simulink model "MPPT_pv_system"  (R2020a)
settings: Solver=VariableStepAuto  StartTime=0.0  StopTime=1  RelTol=1e-3
libraries: powerlib x18, re_lib x1, simulink x1
settings Model: Creator=hp  LastModifiedBy=hp

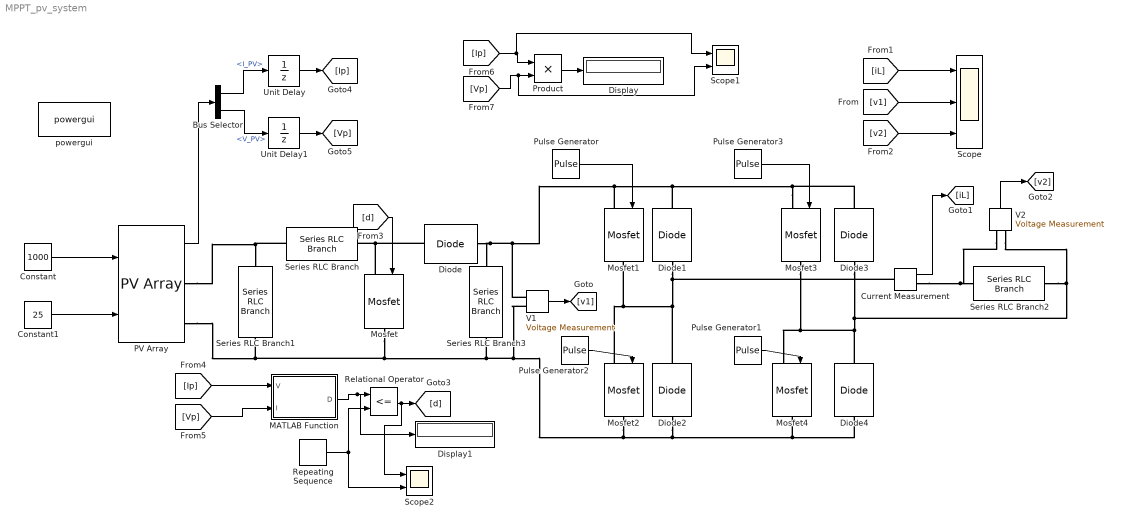
== system MPPT_pv_system ==
  Bus Selector : BusSelector  OutputSignals=I_PV,V_PV
  Constant : Constant  Value=1000
  Constant1 : Constant  Value=25
  Current Measurement : powerlib/Measurements/Current Measurement  PhasorSimulation=off  OutputType=Complex  PSBequivalent=0
  Diode{,1..4} (5 alike) : powerlib/Power Electronics/Diode  Ron=0.001  Lon=0  Vf=0.8  IC=0  UseSnubber=0  Rs=500  Cs=250e-9  Measurements=off
  Display : Display
  Display1 : Display
  MATLAB Function : MATLAB Function  TreatAsAtomicUnit=on
  Mosfet{,1..4} (5 alike) : powerlib/Power Electronics/Mosfet  Ron=0.1  Lon=0  Rd=0.01  Vfd=0  IC=0  Rs=1e5  Cs=inf  Measurements=off
  PV Array : re_lib/Solar/PV Array  Npar=4  Nser=4  PlotType=array @ 25 deg.C & specified irradiances  S_vec="[ 1000  500  100 ]"  Temp_C_vec="[ 45 25  ]"  ModuleName=Centrosolar America BP7-315BW  PlotWhenSelected=off  Pm=315.0042  Ncell=72  Voc=45.45  Isc=8.97  Vm=37.59  Im=8.38  beta_Voc_pc=-0.349  alpha_Isc_pc=0.037001  beta_Voc=-0.15862  alpha_Isc=0.003319  IL=8.9803  I0=1.9823e-10  nI=1.0022  Rsh=237.0635  Rs=0.27147  RobustModel=off  RobustCellTemperature=25  BAL=on  Tc=1e-6  Tfilter=5e-5
  Product : Product
  Pulse Generator : DiscretePulseGenerator  PulseType=Time based  Period=1/(50)  PulseWidth=50  PhaseDelay=0/(360*50)
  Pulse Generator1 : DiscretePulseGenerator  PulseType=Time based  Period=1/(50)  PulseWidth=50  PhaseDelay=0/(360*50)
  Pulse Generator2 : DiscretePulseGenerator  PulseType=Time based  Period=1/(50)  PulseWidth=50  PhaseDelay=180/(360*50)
  Pulse Generator3 : DiscretePulseGenerator  PulseType=Time based  Period=1/(50)  PulseWidth=50  PhaseDelay=180/(360*50)
  Relational Operator : RelationalOperator  Operator=<=  OutDataTypeStr=boolean  RndMeth=Simplest
  Repeating Sequence : simulink/Sources/Repeating Sequence  rep_seq_t=[0 1/(50e3) 2/(50e3)]  rep_seq_y=[0 1 0]
  Scope : Scope  NumInputPorts=3
  Scope1 : Scope  NumInputPorts=2
  Scope2 : Scope  NumInputPorts=2
  Series RLC Branch : powerlib/Elements/Series RLC Branch  LConnTagsString=__new0  RConnTagsString=__new0  BranchType=L  Resistance=1  Inductance=20e-3  SetiL0=off  InitialCurrent=0  Capacitance=1e-6  Setx0=off  InitialVoltage=0  Measurements=None
  Series RLC Branch1 : powerlib/Elements/Series RLC Branch  LConnTagsString=__new0  RConnTagsString=__new0  BranchType=C  Resistance=1  Inductance=1e-3  SetiL0=off  InitialCurrent=0  Capacitance=6e-6  Setx0=off  InitialVoltage=0  Measurements=None
  Series RLC Branch2 : powerlib/Elements/Series RLC Branch  LConnTagsString=__new0  RConnTagsString=__new0  BranchType=R  Resistance=181  Inductance=1e-3  SetiL0=off  InitialCurrent=0  Capacitance=1e-6  Setx0=off  InitialVoltage=0  Measurements=None
  Series RLC Branch3 : powerlib/Elements/Series RLC Branch  LConnTagsString=__new0  RConnTagsString=__new0  BranchType=C  Resistance=1  Inductance=1e-3  SetiL0=off  InitialCurrent=0  Capacitance=64e-6  Setx0=off  InitialVoltage=0  Measurements=None
  Unit Delay : UnitDelay  SampleTime=1e-4  HasFrameUpgradeWarning=on
  Unit Delay1 : UnitDelay  SampleTime=1e-4  HasFrameUpgradeWarning=on
  V1 : powerlib/Measurements/Voltage Measurement  PhasorSimulation=off  OutputType=Complex  PSBequivalent=0
  V2 : powerlib/Measurements/Voltage Measurement  PhasorSimulation=off  OutputType=Complex  PSBequivalent=0
  powergui : powerlib/powergui  Priority=1  SimulationMode=Discrete  SampleTime=50e-8  frequency=60  Iterations=50  frequencyindice=0  Pbase=100e6  ErrMax=1e-4  UnitsV=kV  UnitsW=MW  buscounter=0  FunctionMessages=off  echomessages=off  EnableUseOfTLC=off  CurrentSourceSwitches=off  DisableSnubberDevices=off  DisableRonSwitches=off  DisableVfSwitches=off  DisplayEquations=off  AutomaticDiscreteSolvers=off  SolverType=Tustin/Backward Euler (TBE)  Interpol=off  ExternalGateDelay=off  methode=off  Ts=100  x0status=blocks  SPID=on  SwTol=0  HookPort=off  NonlinearTolerance=1e-4  nMaxIteration=100  ContinueOnMaxIteration=off  RestoreLinks=warning  ResistiveCurrentMeasurement=off  Frange=[0:2:500]  Ylog=off  Xlog=on  ShowGrid=off  save=off  variable=ZData  structure=0  ZoomFFT=off  StartTime=0.0  cycles=1  DisplayStyle=1  fundamental=60  FreqAxis=off  MaxFrequency=1000  frequencyindicesteady=1  RmsSteady=1  display=off
  wires:
  Pulse Generator2/1 -> Mosfet2/1
  Pulse Generator3/1 -> Mosfet3/1
  [iL] -> Scope/1
  V1/1 -> [v1]
  Pulse Generator1/1 -> Mosfet4/1
  Constant1/1 -> PV Array/2
  V2/1 -> [v2]
  [v2] -> Scope/3
  Current Measurement/1 -> [iL]
  [v1] -> Scope/2
  [d] -> Mosfet/1
  Constant/1 -> PV Array/1
  Pulse Generator/1 -> Mosfet1/1
  Product/1 -> Display/1
  MATLAB Function/1(D) -> Display1/1, Relational Operator/1
  Repeating Sequence/1 -> Relational Operator/2, Scope2/2
  Relational Operator/1 -> Scope2/1, [d]
  Unit Delay1/1 -> [Vp]
  Unit Delay/1 -> [Ip]
  PV Array/1 -> Bus Selector/1
  Bus Selector/1 -> Unit Delay/1  "<I_PV>"
  Bus Selector/2 -> Unit Delay1/1  "<V_PV>"
  [Vp] -> Scope1/2, Product/2
  [Ip] -> Scope1/1, Product/1
  [Ip] -> MATLAB Function/1(V)
  [Vp] -> MATLAB Function/2(I)
  connections:
  Mosfet3/LConn1 -- Diode3/RConn1 -- Diode/RConn1 -- Series RLC Branch3/LConn1 -- V1/LConn1 -- Mosfet1/LConn1 -- Diode1/RConn1
  Diode2/RConn1 -- Current Measurement/LConn1 -- Diode1/LConn1 -- Mosfet2/LConn1 -- Mosfet1/RConn1
  Series RLC Branch/LConn1 -- PV Array/RConn1 -- Series RLC Branch1/LConn1
  V1/LConn2 -- Series RLC Branch1/RConn1 -- PV Array/RConn2 -- Mosfet/RConn1 -- Series RLC Branch3/RConn1 -- Diode2/LConn1 -- Diode4/LConn1 -- Mosfet4/RConn1 -- Mosfet2/RConn1
  Current Measurement/RConn1 -- V2/LConn1 -- Series RLC Branch2/LConn1
  Series RLC Branch/RConn1 -- Mosfet/LConn1 -- Diode/LConn1
  Diode3/LConn1 -- V2/LConn2 -- Series RLC Branch2/RConn1 -- Diode4/RConn1 -- Mosfet3/RConn1 -- Mosfet4/LConn1

== matlab function MPPT_pv_system/MATLAB Function ==
  data: V input; D output; I input
function D = Duty_cycle(V,I)
Dmax=.8429;
Dmim=.3675;
Dinit=.8429;
DelD=.0001;
persistent Vold Pold Dold;
datatype='double';

if isempty(Vold)
    Vold = 0;
    Pold = 0;
    Dold = Dinit;
end
P=V*I;
dV=V-Vold;
dP=P-Pold;
if dP~=0; % dP is not equel to zero
 if dP<0;
     if dV<0;
       D=Dold-DelD;
     else
       D=Dold+DelD;
     end
 else
     if dV<0;
       D=Dold+DelD;
     else
       D=Dold-DelD;
     end 
 end
else 
    D=Dold;
end
if D>=Dmax || D<Dmim
    D=Dold;
end
Dold=D;
Vold=V;
Pold=P;
